simulink library "tinbot"  (R2016a)
settings: Solver=ode45  StartTime=0.0  StopTime=10.0  RelTol=1e-3
libraries: tinbot x28, simulink x3
settings Model: Creator=maximilian  LastModifiedBy=maximilian
settings DataIOCC: LimitDataPoints=on
settings DebuggingCC: AllowSymbolicDim=off

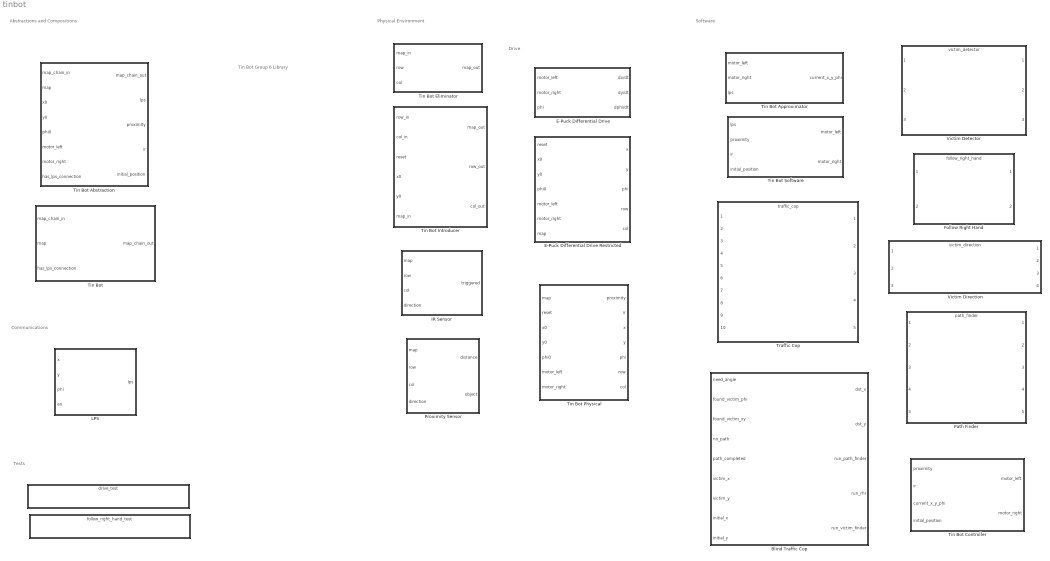
== system tinbot ==
  note: Tests
  note: Abstractions and Compositions
  note: Tin Bot
      | Group 6
      |
      | Library
  note: Communications
  note: Physical Environment
  note: Software
  note: Drive
  " " : ModelReference  ModelNameDialog=drive_test.slx  SimulationMode=Normal  ModelReferenceVersion=1.6
      mask init:
      | pos    = get_param(gcb, 'Position');
      | width  = pos(3) - pos(1);
      | height = pos(4) - pos(2);
      | 
      | 
      | % Compute arrow coordinates
      | arrowW = width  / 20;
      | arrowH = height / 2.5;
      | arrowX = width  / 50;
      | arrowY = height / 3;
      | arrowXvec = [arrowX, arrowX, arrowX + arrowW];
      | arrowYvec = [arrowY, arrowY + arrowH, arrowY + arrowH / 2];
      | 
      | % Compute text position
      | textXbuff = width / 30;
      | textX  = arrowX + arrowW + textXbuff;
      | textY  = height / 2;
      mask Display:
      | patch(arrowXvec, arrowYvec);
      | text(textX, textY, 'Drive Test');
  "  " : ModelReference  ModelNameDialog=follow_right_hand_test.slx  SimulationMode=Normal  ModelReferenceVersion=1.48
      mask init: same as tinbot/ 
      mask Display:
      | patch(arrowXvec, arrowYvec);
      | text(textX, textY, 'Right Hand Rule Test');
  Blind Traffic Cop : Subsystem
      mask Display: fprintf('Tin Bot\nBlind Traffic Cop')
  E-Puck Differential Drive : Subsystem  TreatAsAtomicUnit=on
      mask Display: fprintf('E-Puck\nDifferential Drive')
  E-Puck Differential Drive Restricted : Subsystem
      mask Display: fprintf('E-Puck\nDifferential Drive\n(restricted)')
  Follow Right Hand : ModelReference  ModelNameDialog=follow_right_hand.mdl  SimulationMode=Normal  ModelReferenceVersion=1.25
      mask Display: fprintf('Tin Bot\nFollow Right Hand')
  IR Sensor : Subsystem
      mask Display: fprintf('IR Sensor')
  LPS : Subsystem
      mask Display: fprintf('LPS')
  Path Finder : ModelReference  ModelNameDialog=path_finder.mdl  SimulationMode=Normal  ModelReferenceVersion=1.110
      mask Display: fprintf('Tin Bot\nPath Finder')
  Proximity Sensor : Subsystem
      mask Display: fprintf('Proximity Sensor')
  Tin Bot : Subsystem  mask{x0=100, y0=100, phi0=0}
      mask Display: fprintf('Tin Bot')
  Tin Bot Abstraction : Subsystem
      mask Display: fprintf('Tin Bot\n(abstract)')
  Tin Bot Approximator : Subsystem
      mask Display: fprintf('Tin Bot\nApproximator\n(with motor delay)')
  Tin Bot Controller : Subsystem
      mask Display: fprintf('Tin Bot\nController')
  Tin Bot Eliminator : Subsystem
      mask Display: fprintf('Tin Bot\nEliminator')
  Tin Bot Introducer : Subsystem
      mask Display: fprintf('Tin Bot\nIntroducer')
  Tin Bot Physical : Subsystem
      mask Display: fprintf('Tin Bot\nPhysical\n(with motor delay)')
  Tin Bot Software : Subsystem
      mask Display: fprintf('Tin Bot\nSoftware')
  Traffic Cop : ModelReference  ModelNameDialog=traffic_cop.mdl  SimulationMode=Normal  ModelReferenceVersion=1.107
      mask Display: fprintf('Tin Bot\nTraffic Cop')
  Victim Detector : ModelReference  ModelNameDialog=victim_detector.mdl  SimulationMode=Normal  ModelReferenceVersion=1.11
      mask Display: fprintf('Tin Bot\nVictim Detector')
  Victim Direction : ModelReference  ModelNameDialog=victim_direction.mdl  SimulationMode=Normal  ModelReferenceVersion=1.41
      mask Display: fprintf('Tin Bot\nVictim Direction\nCalculator')

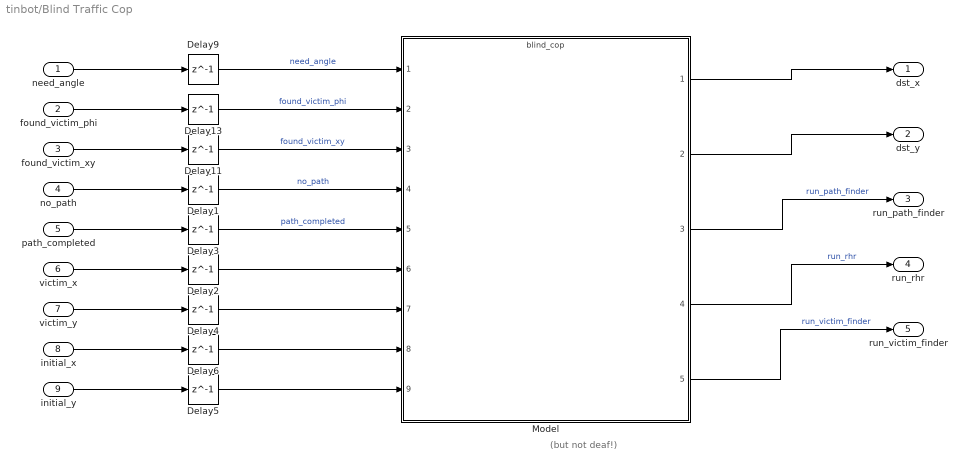
== system tinbot/Blind Traffic Cop ==
  note: (but not deaf!)
  need_angle : Inport
  found_victim_phi : Inport  Port=2
  found_victim_xy : Inport  Port=3
  no_path : Inport  Port=4
  path_completed : Inport  Port=5
  victim_x : Inport  Port=6
  victim_y : Inport  Port=7
  initial_x : Inport  Port=8
  initial_y : Inport  Port=9
  Delay{1..6,9,11,13} (9 alike) : Delay  DelayLength=1
  Model : ModelReference  ModelNameDialog=blind_cop.mdl  SimulationMode=Normal  ModelReferenceVersion=1.103
  dst_x : Outport
  dst_y : Outport  Port=2
  run_path_finder : Outport  Port=3
  run_rhr : Outport  Port=4
  run_victim_finder : Outport  Port=5
  wires:
  Model/5 -> run_victim_finder/1  "run_victim_finder"
  Model/3 -> run_path_finder/1  "run_path_finder"
  Model/4 -> run_rhr/1  "run_rhr"
  Model/2 -> dst_y/1
  Model/1 -> dst_x/1
  found_victim_xy/1 -> Delay11/1
  no_path/1 -> Delay1/1
  found_victim_phi/1 -> Delay13/1
  initial_y/1 -> Delay5/1
  victim_y/1 -> Delay4/1
  victim_x/1 -> Delay2/1
  path_completed/1 -> Delay3/1
  initial_x/1 -> Delay6/1
  need_angle/1 -> Delay9/1
  Delay11/1 -> Model/3  "found_victim_xy"
  Delay6/1 -> Model/8
  Delay4/1 -> Model/7
  Delay9/1 -> Model/1  "need_angle"
  Delay13/1 -> Model/2  "found_victim_phi"
  Delay5/1 -> Model/9
  Delay3/1 -> Model/5  "path_completed"
  Delay1/1 -> Model/4  "no_path"
  Delay2/1 -> Model/6

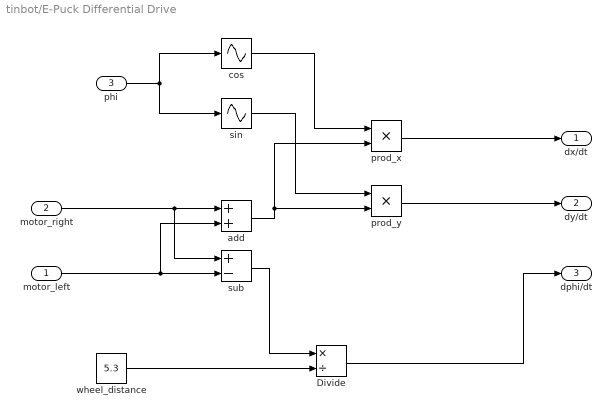
== system tinbot/E-Puck Differential Drive ==
  motor_left : Inport
  motor_right : Inport  Port=2
  phi : Inport  Port=3
  Divide : Product  Inputs=*/
  add : Sum
  cos : Sin  TimeSource=Use external signal  Amplitude=0.5  Phase=pi/2  SampleTime=0
  prod_x : Product
  prod_y : Product
  "sin " : Sin  TimeSource=Use external signal  Amplitude=0.5  SampleTime=0
  sub : Sum  Inputs=+-
  wheel_distance : Constant  Value=5.3
  dx/dt : Outport
  dy/dt : Outport  Port=2
  dphi/dt : Outport  Port=3
  wires:
  motor_left/1 -> sub/2, add/2
  motor_right/1 -> sub/1, add/1
  sub/1 -> Divide/1
  wheel_distance/1 -> Divide/2
  Divide/1 -> dphi/dt/1
  phi/1 -> "sin "/1, cos/1
  add/1 -> prod_x/2, prod_y/2
  "sin "/1 -> prod_y/1
  prod_y/1 -> dy/dt/1
  cos/1 -> prod_x/1
  prod_x/1 -> dx/dt/1

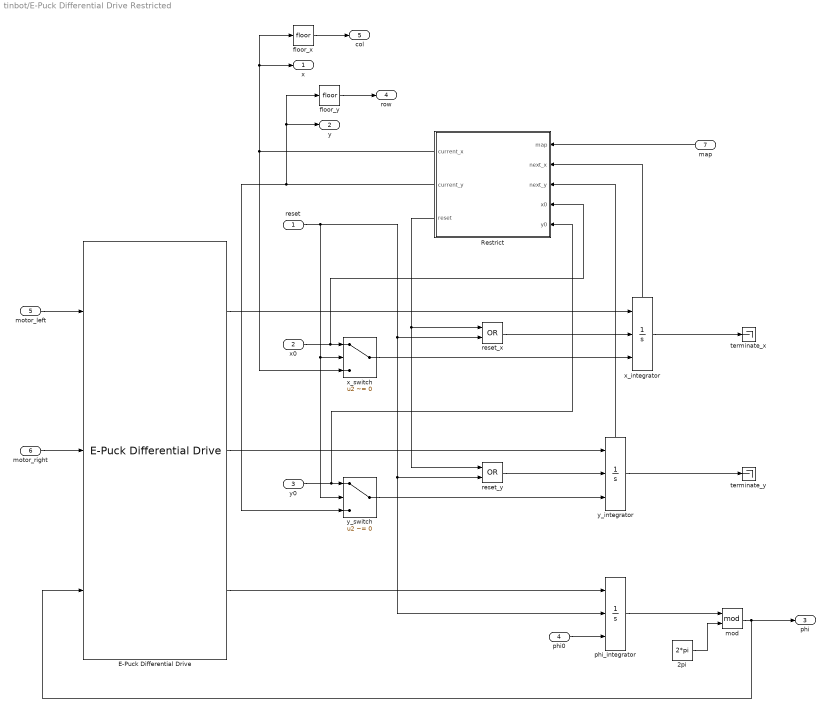
== system tinbot/E-Puck Differential Drive Restricted ==
  reset : Inport
  x0 : Inport  Port=2
  y0 : Inport  Port=3
  phi0 : Inport  Port=4
  motor_left : Inport  Port=5
  motor_right : Inport  Port=6
  map : Inport  Port=7
  2pi : Constant  Value=2*pi
  E-Puck Differential Drive : tinbot/E-Puck Differential Drive  SystemSampleTime=-1
  Restrict : Stateflow chart  TreatAsAtomicUnit=on
  floor_x : Rounding
  floor_y : Rounding
  mod : Math  Operator=mod  SaturateOnIntegerOverflow=on
  phi_integrator : Integrator  ExternalReset=rising  InitialConditionSource=external
  reset_x : Logic  Operator=OR  AllPortsSameDT=off  OutDataTypeStr=boolean
  reset_y : Logic  Operator=OR  AllPortsSameDT=off  OutDataTypeStr=boolean
  terminate_x : Terminator
  terminate_y : Terminator
  x_integrator : Integrator  ExternalReset=rising  InitialConditionSource=external  ShowStatePort=on
  x_switch : Switch  Criteria=u2 ~= 0
  y_integrator : Integrator  ExternalReset=rising  InitialConditionSource=external  ShowStatePort=on
  y_switch : Switch  Criteria=u2 ~= 0
  "x " : Outport
  y : Outport  Port=2
  "phi " : Outport  Port=3
  row : Outport  Port=4
  col : Outport  Port=5
  wires:
  E-Puck Differential Drive/1 -> x_integrator/1
  E-Puck Differential Drive/2 -> y_integrator/1
  E-Puck Differential Drive/3 -> phi_integrator/1
  phi_integrator/1 -> mod/1
  motor_left/1 -> E-Puck Differential Drive/1
  motor_right/1 -> E-Puck Differential Drive/2
  reset_x/1 -> x_integrator/2
  Restrict/3(reset) -> reset_y/1, reset_x/1
  reset_y/1 -> y_integrator/2
  x_switch/1 -> x_integrator/3
  reset/1 -> phi_integrator/2, reset_y/2, reset_x/2, x_switch/2, y_switch/2
  y_switch/1 -> y_integrator/3
  x0/1 -> Restrict/4(x0), x_switch/1
  x_integrator/State -> Restrict/2(next_x)
  y_integrator/State -> Restrict/3(next_y)
  phi0/1 -> phi_integrator/3
  y0/1 -> Restrict/5(y0), y_switch/1
  map/1 -> Restrict/1(map)
  floor_x/1 -> col/1
  Restrict/1(current_x) -> floor_x/1, "x "/1, x_switch/3
  floor_y/1 -> row/1
  Restrict/2(current_y) -> y/1, floor_y/1, y_switch/3
  x_integrator/1 -> terminate_x/1
  y_integrator/1 -> terminate_y/1
  mod/1 -> E-Puck Differential Drive/3, "phi "/1
  2pi/1 -> mod/2

== system tinbot/IR Sensor ==
  map : Inport
  row : Inport  Port=2
  col : Inport  Port=3
  direction : Inport  Port=4
  Sensor : MATLAB Function  TreatAsAtomicUnit=on
  triggered : Outport
  wires:
  map/1 -> Sensor/1(matrix)
  col/1 -> Sensor/3(col)
  row/1 -> Sensor/2(row)
  direction/1 -> Sensor/4(direction)
  Sensor/1(out) -> triggered/1

== system tinbot/LPS ==
  x : Inport
  y : Inport  Port=2
  phi : Inport  Port=3
  en : Inport  Port=4
  Chart : Stateflow chart
  lps : Outport
  wires:
  x/1 -> Chart/1(x)
  y/1 -> Chart/2(y)
  phi/1 -> Chart/3(phi)
  en/1 -> Chart/4(en)
  Chart/1(lps) -> lps/1

== system tinbot/Proximity Sensor ==
  map : Inport
  row : Inport  Port=2
  col : Inport  Port=3
  direction : Inport  Port=4
  Sensor : MATLAB Function  TreatAsAtomicUnit=on
  distance : Outport
  object : Outport  Port=2
  wires:
  map/1 -> Sensor/1(matrix)
  col/1 -> Sensor/3(col)
  row/1 -> Sensor/2(row)
  direction/1 -> Sensor/4(direction)
  Sensor/1(distance) -> distance/1
  Sensor/2(object) -> object/1

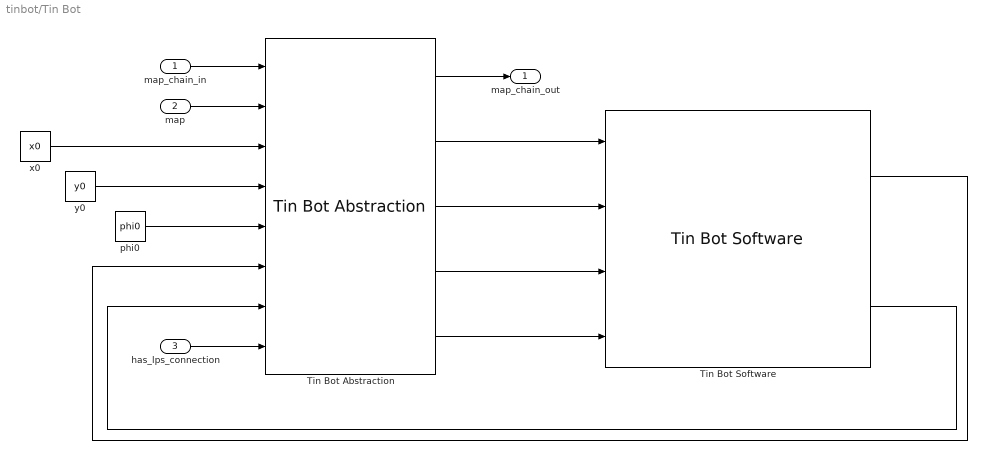
== system tinbot/Tin Bot ==
  map_chain_in : Inport
  map : Inport  Port=2
  has_lps_connection : Inport  Port=3
  Tin Bot Abstraction : tinbot/Tin Bot Abstraction  SystemSampleTime=-1
  Tin Bot Software : tinbot/Tin Bot Software  SystemSampleTime=-1
  phi0 : Constant  Value=phi0
  x0 : Constant  Value=x0
  y0 : Constant  Value=y0
  map_chain_out : Outport
  wires:
  Tin Bot Abstraction/2 -> Tin Bot Software/1
  Tin Bot Abstraction/3 -> Tin Bot Software/2
  Tin Bot Abstraction/4 -> Tin Bot Software/3
  Tin Bot Abstraction/5 -> Tin Bot Software/4
  map/1 -> Tin Bot Abstraction/2
  map_chain_in/1 -> Tin Bot Abstraction/1
  Tin Bot Abstraction/1 -> map_chain_out/1
  x0/1 -> Tin Bot Abstraction/3
  y0/1 -> Tin Bot Abstraction/4
  phi0/1 -> Tin Bot Abstraction/5
  has_lps_connection/1 -> Tin Bot Abstraction/8
  Tin Bot Software/1 -> Tin Bot Abstraction/6
  Tin Bot Software/2 -> Tin Bot Abstraction/7

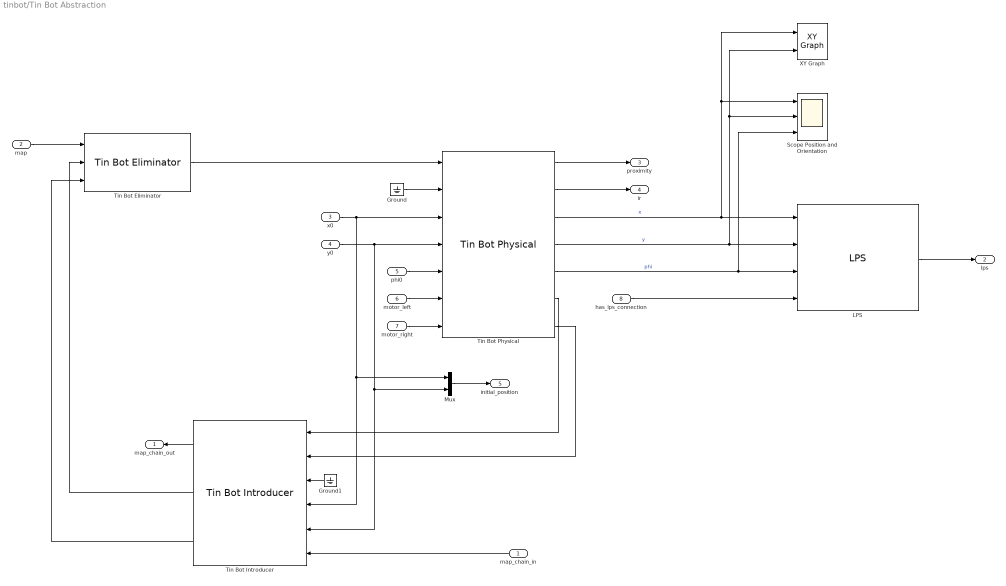
== system tinbot/Tin Bot Abstraction ==
  map_chain_in : Inport
  map : Inport  Port=2
  x0 : Inport  Port=3
  y0 : Inport  Port=4
  phi0 : Inport  Port=5
  motor_left : Inport  Port=6
  motor_right : Inport  Port=7
  has_lps_connection : Inport  Port=8
  Ground : Ground
  Ground1 : Ground
  LPS : tinbot/LPS  SystemSampleTime=-1
  Mux : Mux  Inputs=2
  Scope Position and Orientation : Scope  NumInputPorts=3
  Tin Bot Eliminator : tinbot/Tin Bot Eliminator  SystemSampleTime=-1
  Tin Bot Introducer : tinbot/Tin Bot Introducer  SystemSampleTime=-1
  Tin Bot Physical : tinbot/Tin Bot Physical  SystemSampleTime=-1
  XY Graph : simulink/Sinks/XY Graph  xmin=-1  xmax=1  ymin=-1  ymax=1  st=-1
  map_chain_out : Outport
  lps : Outport  Port=2
  proximity : Outport  Port=3
  ir : Outport  Port=4
  initial_position : Outport  Port=5
  wires:
  Tin Bot Eliminator/1 -> Tin Bot Physical/1
  Tin Bot Physical/6 -> Tin Bot Introducer/1
  Tin Bot Physical/7 -> Tin Bot Introducer/2
  Tin Bot Introducer/3 -> Tin Bot Eliminator/3
  Tin Bot Introducer/2 -> Tin Bot Eliminator/2
  map_chain_in/1 -> Tin Bot Introducer/6
  Tin Bot Introducer/1 -> map_chain_out/1
  map/1 -> Tin Bot Eliminator/1
  y0/1 -> Mux/2, Tin Bot Introducer/5, Tin Bot Physical/4
  Ground/1 -> Tin Bot Physical/2
  Ground1/1 -> Tin Bot Introducer/3
  phi0/1 -> Tin Bot Physical/5
  motor_left/1 -> Tin Bot Physical/6
  motor_right/1 -> Tin Bot Physical/7
  Tin Bot Physical/4 -> XY Graph/2, Scope Position and Orientation/2, LPS/2  "y"
  Tin Bot Physical/5 -> Scope Position and Orientation/3, LPS/3  "phi"
  has_lps_connection/1 -> LPS/4
  LPS/1 -> lps/1
  Tin Bot Physical/1 -> proximity/1
  Tin Bot Physical/2 -> ir/1
  Mux/1 -> initial_position/1
  Tin Bot Physical/3 -> XY Graph/1, Scope Position and Orientation/1, LPS/1  "x"
  x0/1 -> Tin Bot Physical/3, Tin Bot Introducer/4, Mux/1

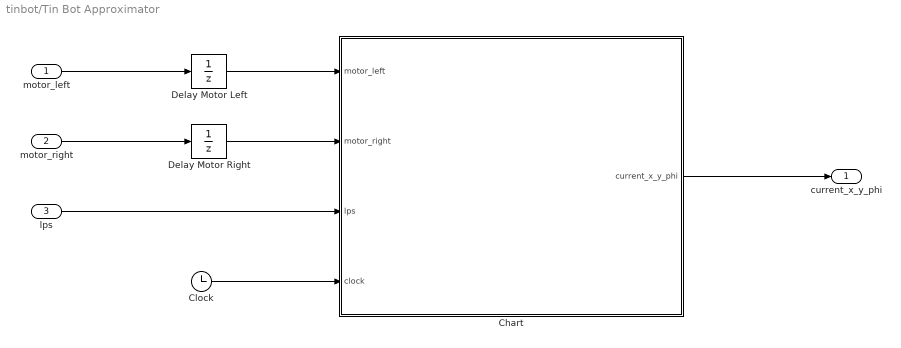
== system tinbot/Tin Bot Approximator ==
  motor_left : Inport
  motor_right : Inport  Port=2
  lps : Inport  Port=3  PortDimensions=[3]
  Chart : Stateflow chart  TreatAsAtomicUnit=on
  Clock : Clock
  Delay Motor Left : UnitDelay  SampleTime=-1
  Delay Motor Right : UnitDelay  SampleTime=-1
  current_x_y_phi : Outport  PortDimensions=[3]
  wires:
  motor_left/1 -> Delay Motor Left/1
  motor_right/1 -> Delay Motor Right/1
  lps/1 -> Chart/3(lps)
  Clock/1 -> Chart/4(clock)
  Chart/1(current_x_y_phi) -> current_x_y_phi/1
  Delay Motor Left/1 -> Chart/1(motor_left)
  Delay Motor Right/1 -> Chart/2(motor_right)

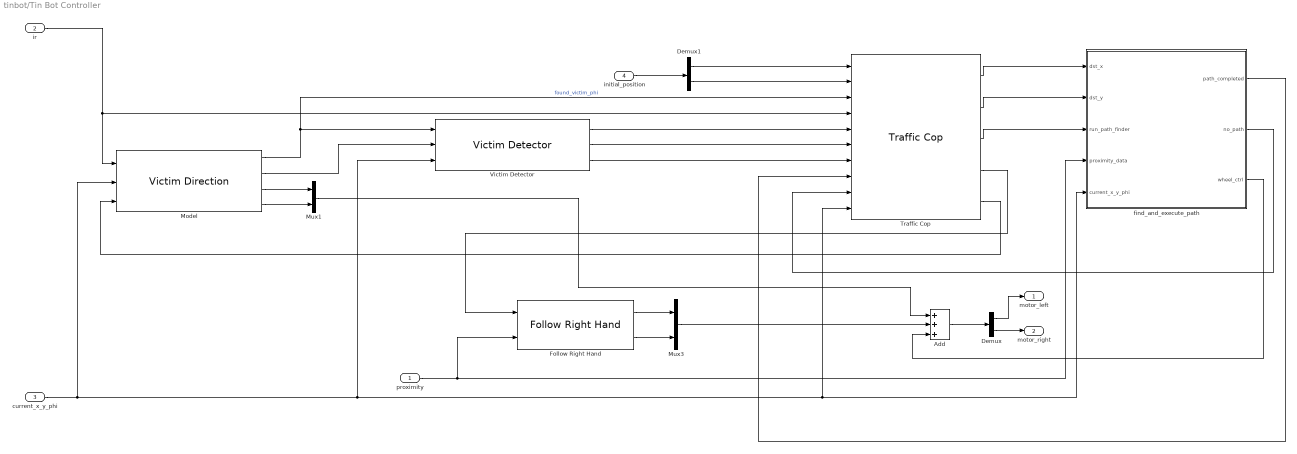
== system tinbot/Tin Bot Controller ==
  proximity : Inport
  ir : Inport  Port=2
  current_x_y_phi : Inport  Port=3
  initial_position : Inport  Port=4
  Add : Sum  Inputs=+++
  Demux : Demux  Outputs=2
  Demux1 : Demux  Outputs=2
  Follow Right Hand : tinbot/Follow Right Hand  SimulationMode=Normal  CodeInterface=Model reference  ModelReferenceVersion=1.25
  Model : tinbot/Victim Direction  SimulationMode=Normal  CodeInterface=Model reference  ModelReferenceVersion=1.41
  Mux1 : Mux  Inputs=2
  Mux3 : Mux  Inputs=2
  Traffic Cop : tinbot/Traffic Cop  SimulationMode=Normal  CodeInterface=Model reference  ModelReferenceVersion=1.107
  Victim Detector : tinbot/Victim Detector  SimulationMode=Normal  CodeInterface=Model reference  ModelReferenceVersion=1.11
  find_and_execute_path : Subsystem
  motor_left : Outport
  motor_right : Outport  Port=2
  wires:
  current_x_y_phi/1 -> Model/2, Victim Detector/3, Traffic Cop/10, find_and_execute_path/5(current_x_y_phi)
  proximity/1 -> Follow Right Hand/2, find_and_execute_path/4(proximity_data)
  ir/1 -> Traffic Cop/4, Model/1
  Mux1/1 -> Add/1
  Mux3/1 -> Add/2
  Follow Right Hand/2 -> Mux3/2
  Follow Right Hand/1 -> Mux3/1
  initial_position/1 -> Demux1/1
  Victim Detector/1 -> Traffic Cop/5
  Victim Detector/2 -> Traffic Cop/6
  Traffic Cop/5 -> Model/3
  Demux1/2 -> Traffic Cop/2
  Demux1/1 -> Traffic Cop/1
  Traffic Cop/3 -> find_and_execute_path/3(run_path_finder)
  Victim Detector/3 -> Traffic Cop/7
  Add/1 -> Demux/1
  Demux/1 -> motor_left/1
  Demux/2 -> motor_right/1
  Traffic Cop/1 -> find_and_execute_path/1(dst_x)
  Traffic Cop/2 -> find_and_execute_path/2(dst_y)
  Traffic Cop/4 -> Follow Right Hand/1
  find_and_execute_path/2(no_path) -> Traffic Cop/9
  find_and_execute_path/3(wheel_ctrl) -> Add/3
  find_and_execute_path/1(path_completed) -> Traffic Cop/8
  Model/3 -> Mux1/1
  Model/4 -> Mux1/2
  Model/2 -> Victim Detector/2
  Model/1 -> Victim Detector/1, Traffic Cop/3  "found_victim_phi"

== system tinbot/Tin Bot Eliminator ==
  map_in : Inport
  row : Inport  Port=2
  col : Inport  Port=3
  Tin Bot Eliminator : MATLAB Function  TreatAsAtomicUnit=on
  map_out : Outport  PortDimensions=[200 200]
  wires:
  map_in/1 -> Tin Bot Eliminator/1(map_in)
  row/1 -> Tin Bot Eliminator/2(row)
  col/1 -> Tin Bot Eliminator/3(col)
  Tin Bot Eliminator/1(map_out) -> map_out/1

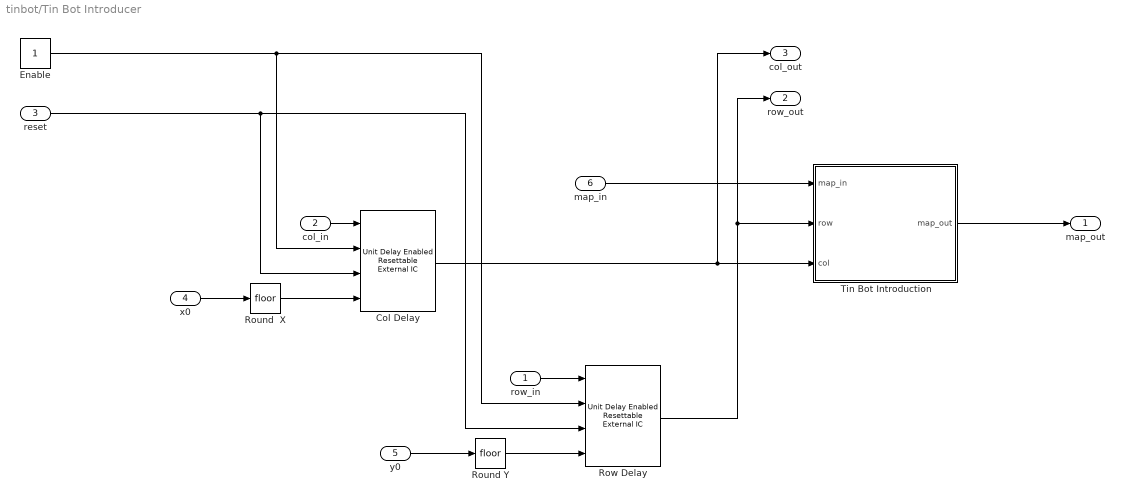
== system tinbot/Tin Bot Introducer ==
  row_in : Inport  Interpolate=off
  col_in : Inport  Port=2  Interpolate=off
  reset : Inport  Port=3
  x0 : Inport  Port=4
  y0 : Inport  Port=5
  map_in : Inport  Port=6  Interpolate=off
  Col Delay : simulink/Additional Math & Discrete/Additional Discrete/Unit Delay Enabled Resettable External IC  tsamp=-1
  Enable : Constant
  Round  X : Rounding
  Round Y : Rounding
  Row Delay : simulink/Additional Math & Discrete/Additional Discrete/Unit Delay Enabled Resettable External IC  tsamp=-1
  Tin Bot Introduction : MATLAB Function  TreatAsAtomicUnit=on
  map_out : Outport
  row_out : Outport  Port=2
  col_out : Outport  Port=3
  wires:
  reset/1 -> Row Delay/3, Col Delay/3
  y0/1 -> Round Y/1
  Round Y/1 -> Row Delay/4
  Round  X/1 -> Col Delay/4
  x0/1 -> Round  X/1
  Enable/1 -> Row Delay/2, Col Delay/2
  col_in/1 -> Col Delay/1
  row_in/1 -> Row Delay/1
  Col Delay/1 -> col_out/1, Tin Bot Introduction/3(col)
  Row Delay/1 -> row_out/1, Tin Bot Introduction/2(row)
  map_in/1 -> Tin Bot Introduction/1(map_in)
  Tin Bot Introduction/1(map_out) -> map_out/1

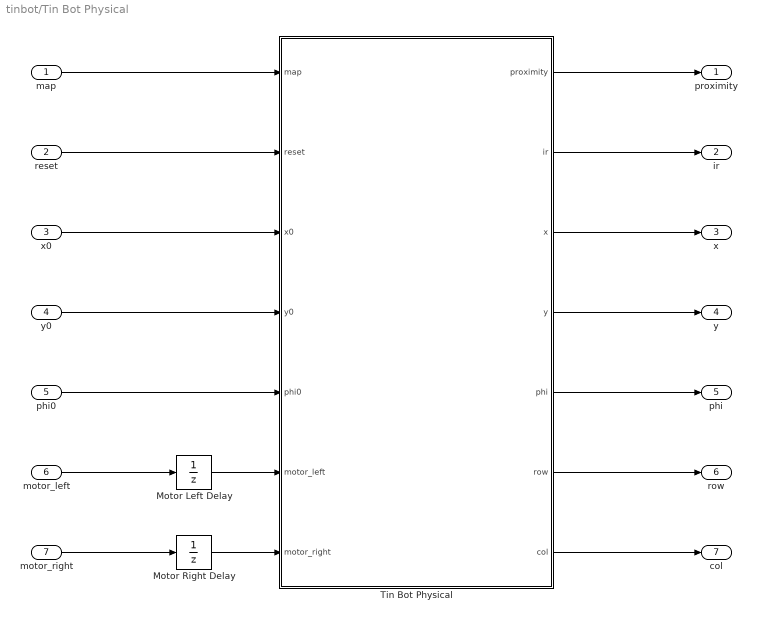
== system tinbot/Tin Bot Physical ==
  map : Inport
  reset : Inport  Port=2
  x0 : Inport  Port=3
  y0 : Inport  Port=4
  phi0 : Inport  Port=5
  motor_left : Inport  Port=6
  motor_right : Inport  Port=7
  Motor Left Delay : UnitDelay  SampleTime=-1
  Motor Right Delay : UnitDelay  SampleTime=-1
  Tin Bot Physical : Subsystem  TreatAsAtomicUnit=on
  proximity : Outport
  ir : Outport  Port=2
  x : Outport  Port=3
  y : Outport  Port=4
  phi : Outport  Port=5
  row : Outport  Port=6
  col : Outport  Port=7
  wires:
  Motor Left Delay/1 -> Tin Bot Physical/6(motor_left)
  Motor Right Delay/1 -> Tin Bot Physical/7(motor_right)
  map/1 -> Tin Bot Physical/1(map)
  reset/1 -> Tin Bot Physical/2(reset)
  x0/1 -> Tin Bot Physical/3(x0)
  y0/1 -> Tin Bot Physical/4(y0)
  phi0/1 -> Tin Bot Physical/5(phi0)
  motor_left/1 -> Motor Left Delay/1
  motor_right/1 -> Motor Right Delay/1
  Tin Bot Physical/1(proximity) -> proximity/1
  Tin Bot Physical/2(ir) -> ir/1
  Tin Bot Physical/3(x) -> x/1
  Tin Bot Physical/4(y) -> y/1
  Tin Bot Physical/5(phi) -> phi/1
  Tin Bot Physical/6(row) -> row/1
  Tin Bot Physical/7(col) -> col/1

== system tinbot/Tin Bot Software ==
  lps : Inport
  proximity : Inport  Port=2
  ir : Inport  Port=3
  initial_position : Inport  Port=4
  Tin Bot Approximator : tinbot/Tin Bot Approximator  SystemSampleTime=-1
  Tin Bot Controller : tinbot/Tin Bot Controller  SystemSampleTime=-1
  motor_left : Outport
  motor_right : Outport  Port=2
  wires:
  lps/1 -> Tin Bot Approximator/3
  proximity/1 -> Tin Bot Controller/1
  ir/1 -> Tin Bot Controller/2
  initial_position/1 -> Tin Bot Controller/4
  Tin Bot Approximator/1 -> Tin Bot Controller/3
  Tin Bot Controller/1 -> motor_left/1, Tin Bot Approximator/1
  Tin Bot Controller/2 -> motor_right/1, Tin Bot Approximator/2

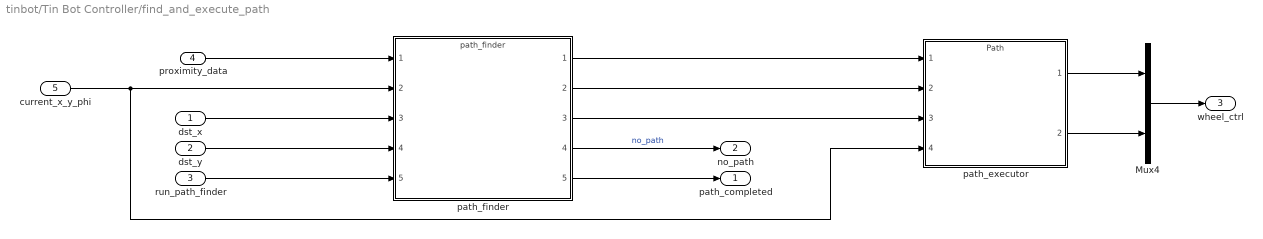
== system tinbot/Tin Bot Controller/find_and_execute_path ==
  dst_x : Inport
  dst_y : Inport  Port=2
  run_path_finder : Inport  Port=3
  proximity_data : Inport  Port=4
  current_x_y_phi : Inport  Port=5
  Mux4 : Mux  Inputs=2
  path_executor : ModelReference  ModelNameDialog=Path.slx  SimulationMode=Normal  ModelReferenceVersion=1.25
  path_finder : ModelReference  ModelNameDialog=path_finder  SimulationMode=Normal  ModelReferenceVersion=1.110
  path_completed : Outport
  no_path : Outport  Port=2
  wheel_ctrl : Outport  Port=3
  wires:
  proximity_data/1 -> path_finder/1
  current_x_y_phi/1 -> path_finder/2, path_executor/4
  path_finder/3 -> path_executor/3
  Mux4/1 -> wheel_ctrl/1
  dst_y/1 -> path_finder/4
  path_finder/4 -> no_path/1  "no_path"
  path_finder/2 -> path_executor/2
  path_finder/1 -> path_executor/1
  run_path_finder/1 -> path_finder/5
  path_executor/2 -> Mux4/2
  dst_x/1 -> path_finder/3
  path_executor/1 -> Mux4/1
  path_finder/5 -> path_completed/1

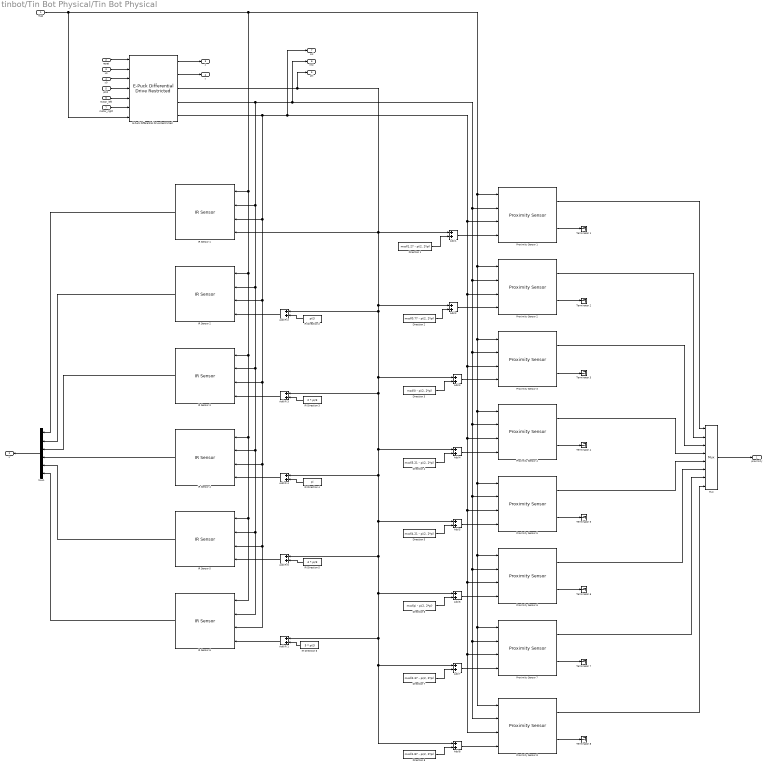
== system tinbot/Tin Bot Physical/Tin Bot Physical ==
  map : Inport
  reset : Inport  Port=2
  x0 : Inport  Port=3
  y0 : Inport  Port=4
  phi0 : Inport  Port=5
  motor_left : Inport  Port=6
  motor_right : Inport  Port=7
  Add {1..8} (8 alike) : Sum
  Add IR {1..5} (5 alike) : Sum
  Direction 1 : Constant  Value=mod(1.27 - pi/2, 2*pi)
  Direction 2 : Constant  Value=mod(0.77 - pi/2, 2*pi)
  Direction 3 : Constant  Value=mod(0 - pi/2, 2*pi)
  Direction 4 : Constant  Value=mod(5.21 - pi/2, 2*pi)
  Direction 5 : Constant  Value=mod(4.21 - pi/2, 2*pi)
  Direction 6 : Constant  Value=mod(pi - pi/2, 2*pi)
  Direction 7 : Constant  Value=mod(2.37 - pi/2, 2*pi)
  Direction 8 : Constant  Value=mod(1.87 - pi/2, 2*pi)
  E-Puck Differential Drive Restricted : tinbot/E-Puck Differential Drive Restricted  SystemSampleTime=-1
  IR Direction 2 : Constant  Value=pi/3
  IR Direction 3 : Constant  Value=2 * pi/3
  IR Direction 4 : Constant  Value=pi
  IR Direction 5 : Constant  Value=4 * pi/3
  IR Direction 6 : Constant  Value=5 * pi/3
  IR Sensor {1..6} (6 alike) : tinbot/IR Sensor  SystemSampleTime=-1
  Mux : Mux  Inputs=8
  Mux1 : Mux  Inputs=6
  Proximity Sensor {1..8} (8 alike) : tinbot/Proximity Sensor  SystemSampleTime=-1
  Terminator {1..8} (8 alike) : Terminator
  proximity : Outport  PortDimensions=8
  ir : Outport  Port=2  PortDimensions=6
  x : Outport  Port=3
  y : Outport  Port=4
  phi : Outport  Port=5
  row : Outport  Port=6
  col : Outport  Port=7
  wires:
  map/1 -> E-Puck Differential Drive Restricted/7, Proximity Sensor 1/1, Proximity Sensor 2/1, Proximity Sensor 3/1, Proximity Sensor 4/1, Proximity Sensor 5/1, Proximity Sensor 6/1, Proximity Sensor 8/1, Proximity Sensor 7/1, IR Sensor 1/1, IR Sensor 2/1, IR Sensor 3/1, IR Sensor 4/1, IR Sensor 6/1, IR Sensor 5/1
  Add 1/1 -> Proximity Sensor 1/4
  Direction 1/1 -> Add 1/2
  Add 2/1 -> Proximity Sensor 2/4
  Direction 2/1 -> Add 2/2
  Add 3/1 -> Proximity Sensor 3/4
  Direction 3/1 -> Add 3/2
  Add 4/1 -> Proximity Sensor 4/4
  Direction 4/1 -> Add 4/2
  Add 5/1 -> Proximity Sensor 5/4
  Direction 5/1 -> Add 5/2
  Add 6/1 -> Proximity Sensor 6/4
  Direction 6/1 -> Add 6/2
  Add 7/1 -> Proximity Sensor 7/4
  Direction 7/1 -> Add 7/2
  Add 8/1 -> Proximity Sensor 8/4
  Direction 8/1 -> Add 8/2
  E-Puck Differential Drive Restricted/4 -> row/1, Proximity Sensor 1/2, Proximity Sensor 2/2, Proximity Sensor 3/2, Proximity Sensor 4/2, Proximity Sensor 5/2, Proximity Sensor 6/2, Proximity Sensor 8/2, Proximity Sensor 7/2, IR Sensor 1/2, IR Sensor 2/2, IR Sensor 3/2, IR Sensor 4/2, IR Sensor 6/2, IR Sensor 5/2
  Proximity Sensor 1/1 -> Mux/1
  Proximity Sensor 2/1 -> Mux/2
  Proximity Sensor 3/1 -> Mux/3
  Proximity Sensor 4/1 -> Mux/4
  Proximity Sensor 5/1 -> Mux/5
  Proximity Sensor 6/1 -> Mux/6
  Proximity Sensor 7/1 -> Mux/7
  Proximity Sensor 8/1 -> Mux/8
  Mux/1 -> proximity/1
  E-Puck Differential Drive Restricted/3 -> phi/1, IR Sensor 1/4, Add 8/1, Add 7/1, Add IR 1/1, Add 6/1, Add IR 5/1, Add 5/1, Add IR 4/1, Add 4/1, Add IR 3/1, Add 3/1, Add IR 2/1, Add 2/1, Add 1/1
  Add IR 2/1 -> IR Sensor 2/4
  IR Direction 2/1 -> Add IR 2/2
  IR Direction 3/1 -> Add IR 3/2
  Add IR 3/1 -> IR Sensor 3/4
  IR Direction 4/1 -> Add IR 4/2
  Add IR 4/1 -> IR Sensor 4/4
  Add IR 5/1 -> IR Sensor 5/4
  IR Direction 5/1 -> Add IR 5/2
  Add IR 1/1 -> IR Sensor 6/4
  IR Direction 6/1 -> Add IR 1/2
  IR Sensor 1/1 -> Mux1/1
  IR Sensor 2/1 -> Mux1/2
  IR Sensor 3/1 -> Mux1/3
  IR Sensor 4/1 -> Mux1/4
  IR Sensor 5/1 -> Mux1/5
  Mux1/1 -> ir/1
  Proximity Sensor 5/2 -> Terminator 5/1
  Proximity Sensor 6/2 -> Terminator 6/1
  Proximity Sensor 4/2 -> Terminator 4/1
  Proximity Sensor 3/2 -> Terminator 3/1
  Proximity Sensor 2/2 -> Terminator 2/1
  Proximity Sensor 1/2 -> Terminator 1/1
  Proximity Sensor 7/2 -> Terminator 7/1
  Proximity Sensor 8/2 -> Terminator 8/1
  E-Puck Differential Drive Restricted/1 -> x/1
  E-Puck Differential Drive Restricted/2 -> y/1
  E-Puck Differential Drive Restricted/5 -> IR Sensor 1/3, IR Sensor 2/3, IR Sensor 3/3, IR Sensor 4/3, IR Sensor 6/3, IR Sensor 5/3, col/1, Proximity Sensor 1/3, Proximity Sensor 2/3, Proximity Sensor 3/3, Proximity Sensor 4/3, Proximity Sensor 5/3, Proximity Sensor 6/3, Proximity Sensor 8/3, Proximity Sensor 7/3
  reset/1 -> E-Puck Differential Drive Restricted/1
  x0/1 -> E-Puck Differential Drive Restricted/2
  y0/1 -> E-Puck Differential Drive Restricted/3
  phi0/1 -> E-Puck Differential Drive Restricted/4
  motor_left/1 -> E-Puck Differential Drive Restricted/5
  motor_right/1 -> E-Puck Differential Drive Restricted/6
  IR Sensor 6/1 -> Mux1/6

== matlab function tinbot/Tin Bot Eliminator/Tin Bot Eliminator ==
  data: map_in input; map_out output; row input; col input
function map_out = eliminate(map_in, row, col)
    map_in(row-2, col) = 0;
    
    map_in(row-1, col-1) = 0;
    map_in(row-1, col) = 0;
    map_in(row-1, col+1) = 0;
    
    map_in(row, col+2) = 0;
    map_in(row, col+1) = 0;
    map_in(row, col) = 0;
    map_in(row, col-1) = 0;
    map_in(row, col-2) = 0;
    
    map_in(row+1, col-1) = 0;
    map_in(row+1, col) = 0;
    map_in(row+1, col+1) = 0;
    
    map_in(row+2, col) = 0;
    
    map_out = map_in;

== matlab function tinbot/Tin Bot Introducer/Tin Bot Introduction ==
  data: map_in input; map_out output; row input; col input
function map_out = introduce(map_in, row, col)
    map_in(row-2, col) = 3;
    
    map_in(row-1, col-1) = 3;
    map_in(row-1, col) = 3;
    map_in(row-1, col+1) = 3;
    
    map_in(row, col+2) = 3;
    map_in(row, col+1) = 3;
    map_in(row, col) = 3;
    map_in(row, col-1) = 3;
    map_in(row, col-2) = 3;
    
    map_in(row+1, col-1) = 3;
    map_in(row+1, col) = 3;
    map_in(row+1, col+1) = 3;
    
    map_in(row+2, col) = 3;
    
    map_out = map_in;

== stateflow chart tinbot/E-Puck Differential Drive Restricted/Restrict ==
  state Start
  state Reset
  (default) -> Start : {
      | 	current_x = x0; current_y = y0; reset = 0;
      | 	x = current_x; y = current_y;
      | 	col = floor(x) + 1; row = floor(y) + 1
      | }
  Start -> Start [order 2] : {
      | 	x = next_x; y = next_y;
      | 	col = floor(y); row = floor(x) ;
      | 	current_x = x;
      | 	current_y = y;
      | }
  Reset -> Start : {reset = 0;}
  Start -> Reset [order 1] : [(floor(next_y) ~= row || floor(next_x) ~= col) && (map(floor(next_y)-2, floor(next_x)) ~= 0 || map(floor(next_y)+2, floor(next_x)) ~= 0 || map(floor(next_y), floor(next_x)-2) ~= 0 || map(floor(next_y), floor(next_x)+2) ~= 0 || map(floor(next_y)+1, floor(next_x)+1) ~= 0 || map(floor(next_y)+1, floor(next_x)-1) ~= 0 || map(floor(next_y)-1, floor(next_x)+1) ~= 0 || map(floor(next_y)-1, floor(next_x)-1) ~= 0)]{
      | 	reset = 1;
      | 	current_x = x;
      | 	current_y = y;
      | }
  data: map input; next_x input; next_y input; current_x output =0; current_y output =0; reset output =0; x local; y local; x0 input; y0 input; col local; row local

== matlab function tinbot/Proximity Sensor/Sensor ==
  data: matrix input; row input; col input; distance output; direction input; object output
function [distance, object] = raycast(matrix, row, col, direction)
    [distance, object] = TinUtils.raycast_polymorphic(matrix, row, col, direction);
    distance =  distance - 2.5;
end

== matlab function tinbot/IR Sensor/Sensor ==
  data: matrix input; row input; col input; out output; direction input
function out  = raycast(matrix, row, col, direction)
    out = 0;
    start = mod(direction - deg2rad(80) / 2, 2 * pi);
    step = deg2rad(80) / 100;
    for i = 0:100
        [~, object] = TinUtils.raycast_polymorphic(matrix, row, col, start + step * i, false);
        if (object == 2)
            out = 1;
            break;
        end
    end
end

== stateflow chart tinbot/LPS/Chart ==
  state Init
  state Start
  state Send
  (default) -> Init : {
      | 	lps = [x; y; phi];
      | }
  Init -> Start : {
      | 	lps = [-1; -1; -1];
      | }
  Send -> Start : {
      | 	lps = [-1; -1; -1];
      | }
  Start -> Send : [after(2, sec) && en == 1] {
      | 	lps = [x; y; phi];
      | }
  data: x input; y input; phi input; en input; lps output

== stateflow chart tinbot/Tin Bot Approximator/Chart ==
  state Update
    during:
    if lps(1) ~= -1
    x = lps(1);
    y = lps(2);
    phi = lps(3);
    else
    v = (prev_motor_left + prev_motor_right) / 2;
    p = (prev_motor_right - prev_motor_left) / 5.3;
    delta_t = clock - prev_t;
    delta_phi = p * delta_t;
    if p == 0
    x = v * cos(phi) * delta_t + x;
    y = v * sin(phi) * delta_t + y;
    else
    x = v * (sin(delta_phi + phi) - sin(phi)) / p + x;
    y = v * (cos(phi) - cos(delta_phi + phi)) / p + y;
    end
    phi = mod(phi + p * delta_t, 2 * pi);
    end
    prev_t = clock;
    prev_motor_left = motor_left;
    prev_motor_right = motor_right;
    current_x_y_phi = [x; y; phi];
  (default) -> Update : {
      | 	x = lps(1);
      | 	y = lps(2);
      | 	phi = lps(3);
      | 	prev_motor_left = 0;
      | 	prev_motor_right = 0;
      | 	prev_t = clock;
      | 	current_x_y_phi = [x; y; phi];
      | }
  data: motor_left input; motor_right input; lps input; clock input; current_x_y_phi output; x local; y local; phi local; v local; prev_motor_left local; p local; delta_t local; prev_t local; delta_phi local; prev_motor_right local
